simulink model "TimxAllConfigurations"  (R2018b)
settings: Solver=FixedStepDiscrete  StartTime=0.0  StopTime=10.0  RelTol=1e-3
libraries: TIMERS_Lib x7, STM32_Config_Lib x1
settings Model: Creator=fenard1  LastModifiedBy=fenard1
settings OptimizationCC: DefaultParameterBehavior=Inlined  DefaultUnderspecifiedDataType=single  EnhancedBackFolding=on  PassReuseOutputArgsAs=Individual arguments  OptimizeBlockOrder=speed  DifferentSizesBufferReuse=on  OptimizationCustomize=off
settings DebuggingCC: ParameterTunabilityLossMsg=error  UniqueDataStoreMsg=error  StrictBusMsg=ErrorOnBusTreatedAsVector  SFUndirectedBroadcastEventsDiag=error
settings HardwareCC: ProdBitPerPointer=32  ProdBitPerSizeT=32  ProdBitPerPtrDiffT=32  ProdLargestAtomicInteger=Integer  ProdWordSize=32  ProdHWDeviceType=STM32CortexM
settings SFSimCC: CompileTimeRecursionLimit=0  EnableRuntimeRecursion=off  MATLABDynamicMemAlloc=off
settings RTWCC: SystemTargetFile=stm32.tlc  TemplateMakefile=stm32.tmf  Description=stm32 (Embedded Target)  GenerateReport=on  IncludeHyperlinkInReport=on
settings CodeAppCC: ForceParamTrailComments=on  IgnoreCustomStorageClasses=off  OperatorAnnotations=on  SimulinkDataObjDesc=on  SFDataObjDesc=on  CustomSymbolStrType=$N$R$M  SimulinkBlockComments=off
settings STFCustomTargetCC: TargetLangStandard=C99 (ISO)  MultiwordLength=256  ParMdlRefBuildCompliant=on  IncludeMdlTerminateFcn=off  CombineOutputUpdateFcns=on  ERTCustomFileBanners=on  SupportComplex=off  SupportContinuousTime=off  SupportNonInlinedSFcns=off  RemoveResetFunc=on  ParenthesesLevel=Maximum  CastingMode=Standards  MATLABClassNameForMDSCustomization=Simulink.SoftwareTarget.ERTCustomization  SystemTargetFile=stm32.tlc
settings ERTTargetCC: TargetLangStandard=C99 (ISO)  CompOptLevelCompliant=off  ConcurrentExecutionCompliant=off  IncludeMdlTerminateFcn=off  SupportComplex=off  ParenthesesLevel=Maximum  CastingMode=Standards  ModelStepFunctionPrototypeControlCompliant=off  CPPClassGenCompliant=off  UseToolchainInfoCompliant=off  ExtModeStaticAllocSize=256  ExtModeMexArgs=0,1,115200,10  InlinedParameterPlacement=NonHierarchical  ERTSrcFileBannerTemplate=sourceFileTemplate.cgt  ERTHdrFileBannerTemplate=sourceFileTemplate.cgt  ERTDataSrcFileTemplate=sourceFileTemplate.cgt  ERTDataHdrFileTemplate=sourceFileTemplate.cgt  ERTCustomFileTemplate=customRoutineProcess.tlc  EnableSignedLeftShifts=off  EnableSignedRightShifts=off

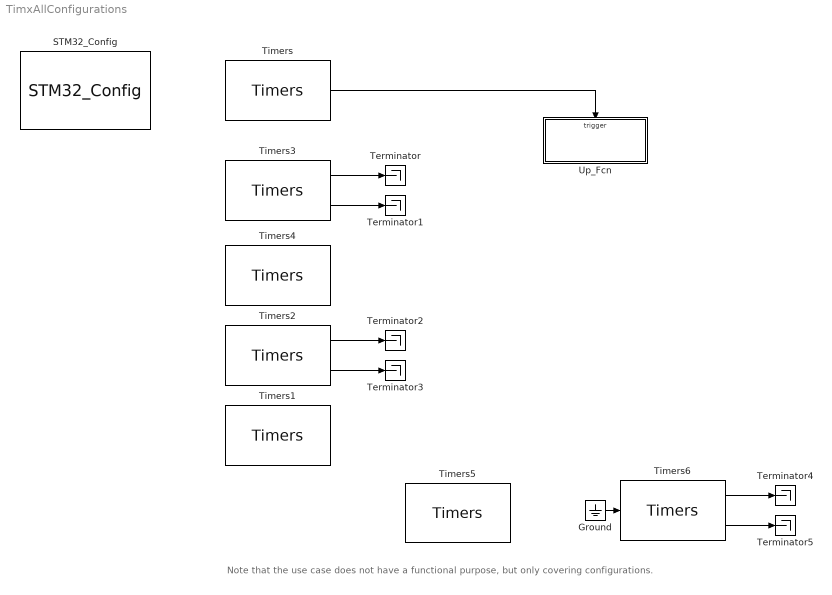
== system TimxAllConfigurations ==
  note: Note that the use case does not have a functional purpose, but only covering configurations.
  Ground : Ground
  STM32_Config : STM32_Config_Lib/STM32_Config  Priority=0  Project_Path=.\  Config_File=TimxAllConfigurations.ioc  MCU_Name=STM32F429ZITx
      settings: SourceProductName=Target Support Package - STM32 Adapter
  Terminator{,1..5} (6 alike) : Terminator
  Timers : TIMERS_Lib/Timers  currentTIM=TIM1  TIM_Name=TIM1  sysUsingTimer=on  TIM_APBClock=180000000  TIM_Set_Clk=off  TIM_Prescaler=2  TIM_Clock=60000000.00  Variable_frequency=off  TIM_Set_OutFreq=off  TIM_ARR=1  Output_frequency=60000000.00  Repetition_counter=0  TIM_Mode=Up  TIM_DMA=none  TIM_IRQ=on  TIM_IRQ_ONLY=off  TIM_UP=on  TIM_TRG=off  TIM_COM=off  TIM_BRK=off  NbTIM=7  CH1_enable=off  CH1N_enable=off  CH1_type=Input_Capture  CH1_DMA=off  CH1_int=off  CH1_edge=Rising  CH1_div=1  CH1_variable_duty=off  CH1_set_pulse=off  CH1_output_duty=0.00  CH1_pulse=0  CH2_enable=on  CH2N_enable=off  CH2_type=Output_Comp  CH2_DMA=off  CH2_int=off  CH2_edge=Rising  CH2_div=1  CH2_variable_duty=off  CH2_set_pulse=off  CH2_output_duty=0.00  CH2_pulse=0  CH3_enable=on  CH3N_enable=on  CH3_type=Output_Comp  CH3_DMA=off  CH3_int=off  CH3_edge=Rising  CH3_div=1  CH3_variable_duty=off  CH3_set_pulse=off  CH3_output_duty=0.00  CH3_pulse=0  CH4_enable=off  CH4N_enable=off  CH4_type=Input_Capture  CH4_DMA=off  CH4_int=off  CH4_edge=Rising  CH4_div=1  CH4_variable_duty=off  CH4_set_pulse=off  CH4_output_duty=0.00  CH4_pulse=0
      settings: SourceProductName=Target Support Package - STM32 Adapter
  Timers1 : TIMERS_Lib/Timers  currentTIM=TIM5  TIM_Name=TIM5  sysUsingTimer=on  TIM_APBClock=90000000  TIM_Set_Clk=off  TIM_Prescaler=0  TIM_Clock=90000000.00  Variable_frequency=off  TIM_Set_OutFreq=off  TIM_ARR=1  Output_frequency=90000000.00  Repetition_counter=0  TIM_Mode=Up  TIM_DMA=none  TIM_IRQ=off  TIM_IRQ_ONLY=on  TIM_UP=off  TIM_TRG=off  TIM_COM=off  TIM_BRK=off  NbTIM=7  CH1_enable=off  CH1N_enable=off  CH1_type=Input_Capture  CH1_DMA=off  CH1_int=off  CH1_edge=Rising  CH1_div=1  CH1_variable_duty=off  CH1_set_pulse=off  CH1_output_duty=0.00  CH1_pulse=0  CH2_enable=on  CH2N_enable=off  CH2_type=Input_Capture  CH2_DMA=off  CH2_int=off  CH2_edge=Rising  CH2_div=1  CH2_variable_duty=off  CH2_set_pulse=off  CH2_output_duty=0.00  CH2_pulse=0  CH3_enable=on  CH3N_enable=off  CH3_type=Output_Comp  CH3_DMA=off  CH3_int=off  CH3_edge=Rising  CH3_div=1  CH3_variable_duty=off  CH3_set_pulse=off  CH3_output_duty=0.00  CH3_pulse=0  CH4_enable=on  CH4N_enable=off  CH4_type=Output_Forced  CH4_DMA=off  CH4_int=off  CH4_edge=Rising  CH4_div=1  CH4_variable_duty=off  CH4_set_pulse=off  CH4_output_duty=0.00  CH4_pulse=0
      settings: SourceProductName=Target Support Package - STM32 Adapter
  Timers2 : TIMERS_Lib/Timers  currentTIM=TIM4  TIM_Name=TIM4  sysUsingTimer=on  TIM_APBClock=90000000  TIM_Set_Clk=off  TIM_Prescaler=0  TIM_Clock=90000000.00  Variable_frequency=off  TIM_Set_OutFreq=off  TIM_ARR=1  Output_frequency=90000000.00  Repetition_counter=0  TIM_Mode=Up  TIM_DMA=none  TIM_IRQ=off  TIM_IRQ_ONLY=off  TIM_UP=off  TIM_TRG=off  TIM_COM=off  TIM_BRK=off  NbTIM=7  CH1_enable=on  CH1N_enable=off  CH1_type=Input_Capture  CH1_DMA=off  CH1_int=off  CH1_edge=Rising  CH1_div=1  CH1_variable_duty=off  CH1_set_pulse=off  CH1_output_duty=0.00  CH1_pulse=0  CH2_enable=on  CH2N_enable=off  CH2_type=Output_Comp  CH2_DMA=off  CH2_int=off  CH2_edge=Rising  CH2_div=1  CH2_variable_duty=off  CH2_set_pulse=off  CH2_output_duty=0.00  CH2_pulse=0  CH3_enable=on  CH3N_enable=off  CH3_type=Output_PWM  CH3_DMA=off  CH3_int=off  CH3_edge=Rising  CH3_div=1  CH3_variable_duty=off  CH3_set_pulse=off  CH3_output_duty=0.00  CH3_pulse=0  CH4_enable=on  CH4N_enable=off  CH4_type=Output_Forced  CH4_DMA=off  CH4_int=off  CH4_edge=Rising  CH4_div=1  CH4_variable_duty=off  CH4_set_pulse=off  CH4_output_duty=0.00  CH4_pulse=0
      settings: SourceProductName=Target Support Package - STM32 Adapter
  Timers3 : TIMERS_Lib/Timers  currentTIM=TIM2  TIM_Name=TIM2  sysUsingTimer=on  TIM_APBClock=90000000  TIM_Set_Clk=off  TIM_Prescaler=0  TIM_Clock=90000000.00  Variable_frequency=off  TIM_Set_OutFreq=off  TIM_ARR=1  Output_frequency=90000000.00  Repetition_counter=0  TIM_Mode=Down  TIM_DMA=none  TIM_IRQ=off  TIM_IRQ_ONLY=off  TIM_UP=off  TIM_TRG=off  TIM_COM=off  TIM_BRK=off  NbTIM=7  CH1_enable=on  CH1N_enable=off  CH1_type=Input_Capture  CH1_DMA=off  CH1_int=off  CH1_edge=Rising  CH1_div=1  CH1_variable_duty=off  CH1_set_pulse=off  CH1_output_duty=0.00  CH1_pulse=0  CH2_enable=off  CH2N_enable=off  CH2_type=Output_PWM  CH2_DMA=off  CH2_int=off  CH2_edge=Rising  CH2_div=1  CH2_variable_duty=off  CH2_set_pulse=off  CH2_output_duty=0.00  CH2_pulse=0  CH3_enable=off  CH3N_enable=off  CH3_type=Output_Forced  CH3_DMA=off  CH3_int=off  CH3_edge=Rising  CH3_div=1  CH3_variable_duty=off  CH3_set_pulse=off  CH3_output_duty=0.00  CH3_pulse=0  CH4_enable=off  CH4N_enable=off  CH4_type=Unknown  CH4_DMA=off  CH4_int=off  CH4_edge=Rising  CH4_div=1  CH4_variable_duty=off  CH4_set_pulse=off  CH4_output_duty=0.00  CH4_pulse=0
      settings: SourceProductName=Target Support Package - STM32 Adapter
  Timers4 : TIMERS_Lib/Timers  currentTIM=TIM3  TIM_Name=TIM3  sysUsingTimer=on  TIM_APBClock=90000000  TIM_Set_Clk=off  TIM_Prescaler=0  TIM_Clock=90000000.00  Variable_frequency=off  TIM_Set_OutFreq=off  TIM_ARR=1  Output_frequency=90000000.00  Repetition_counter=0  TIM_Mode=Center_Aligned_1  TIM_DMA=none  TIM_IRQ=off  TIM_IRQ_ONLY=off  TIM_UP=off  TIM_TRG=off  TIM_COM=off  TIM_BRK=off  NbTIM=7  CH1_enable=off  CH1N_enable=off  CH1_type=Output_Forced  CH1_DMA=off  CH1_int=off  CH1_edge=Rising  CH1_div=1  CH1_variable_duty=off  CH1_set_pulse=off  CH1_output_duty=0.00  CH1_pulse=0  CH2_enable=on  CH2N_enable=off  CH2_type=Output_PWM  CH2_DMA=off  CH2_int=off  CH2_edge=Rising  CH2_div=1  CH2_variable_duty=off  CH2_set_pulse=off  CH2_output_duty=0.00  CH2_pulse=0  CH3_enable=on  CH3N_enable=off  CH3_type=Output_Forced  CH3_DMA=off  CH3_int=off  CH3_edge=Rising  CH3_div=1  CH3_variable_duty=off  CH3_set_pulse=off  CH3_output_duty=0.00  CH3_pulse=0  CH4_enable=off  CH4N_enable=off  CH4_type=Output_PWM  CH4_DMA=off  CH4_int=off  CH4_edge=Rising  CH4_div=1  CH4_variable_duty=off  CH4_set_pulse=off  CH4_output_duty=0.00  CH4_pulse=0
      settings: SourceProductName=Target Support Package - STM32 Adapter
  Timers5 : TIMERS_Lib/Timers  currentTIM=TIM7  TIM_Name=TIM7  sysUsingTimer=on  TIM_APBClock=90000000  TIM_Set_Clk=off  TIM_Prescaler=0  TIM_Clock=90000000.00  Variable_frequency=off  TIM_Set_OutFreq=off  TIM_ARR=1  Output_frequency=90000000.00  Repetition_counter=0  TIM_Mode=Up  TIM_DMA=none  TIM_IRQ=off  TIM_IRQ_ONLY=on  TIM_UP=off  TIM_TRG=off  TIM_COM=off  TIM_BRK=off  NbTIM=7  CH1_enable=off  CH1N_enable=off  CH1_type=Unknown  CH1_DMA=off  CH1_int=off  CH1_edge=Rising  CH1_div=1  CH1_variable_duty=off  CH1_set_pulse=off  CH1_output_duty=0.00  CH1_pulse=0  CH2_enable=off  CH2N_enable=off  CH2_type=Unknown  CH2_DMA=off  CH2_int=off  CH2_edge=Rising  CH2_div=1  CH2_variable_duty=off  CH2_set_pulse=off  CH2_output_duty=0.00  CH2_pulse=0  CH3_enable=off  CH3N_enable=off  CH3_type=Unknown  CH3_DMA=off  CH3_int=off  CH3_edge=Rising  CH3_div=1  CH3_variable_duty=off  CH3_set_pulse=off  CH3_output_duty=0.00  CH3_pulse=0  CH4_enable=off  CH4N_enable=off  CH4_type=Unknown  CH4_DMA=off  CH4_int=off  CH4_edge=Rising  CH4_div=1  CH4_variable_duty=off  CH4_set_pulse=off  CH4_output_duty=0.00  CH4_pulse=0
      settings: SourceProductName=Target Support Package - STM32 Adapter
  Timers6 : TIMERS_Lib/Timers  currentTIM=TIM8  TIM_Name=TIM8  sysUsingTimer=on  TIM_APBClock=180000000  TIM_Set_Clk=off  TIM_Prescaler=0  TIM_Clock=180000000.00  Variable_frequency=off  TIM_Set_OutFreq=off  TIM_ARR=1399  Output_frequency=128663.33  Repetition_counter=0  TIM_Mode=Up  TIM_DMA=none  TIM_IRQ=off  TIM_IRQ_ONLY=off  TIM_UP=off  TIM_TRG=off  TIM_COM=off  TIM_BRK=off  NbTIM=7  CH1_enable=on  CH1N_enable=off  CH1_type=Input_Encoder  CH1_DMA=off  CH1_int=off  CH1_edge=Rising  CH1_div=1  CH1_variable_duty=off  CH1_set_pulse=off  CH1_output_duty=0.00  CH1_pulse=0  CH2_enable=on  CH2N_enable=off  CH2_type=Input_Encoder  CH2_DMA=off  CH2_int=off  CH2_edge=Rising  CH2_div=1  CH2_variable_duty=off  CH2_set_pulse=off  CH2_output_duty=0.00  CH2_pulse=0  CH3_enable=off  CH3N_enable=off  CH3_type=Unknown  CH3_DMA=off  CH3_int=off  CH3_edge=Rising  CH3_div=1  CH3_variable_duty=off  CH3_set_pulse=off  CH3_output_duty=0.00  CH3_pulse=0  CH4_enable=off  CH4N_enable=off  CH4_type=Unknown  CH4_DMA=off  CH4_int=off  CH4_edge=Rising  CH4_div=1  CH4_variable_duty=off  CH4_set_pulse=off  CH4_output_duty=0.00  CH4_pulse=0
      settings: SourceProductName=Target Support Package - STM32 Adapter
  "Up_Fcn " : Subsystem  TreatAsAtomicUnit=on
  wires:
  Timers/1 -> "Up_Fcn "/Trigger
  Timers3/1 -> Terminator/1
  Timers3/2 -> Terminator1/1
  Timers2/1 -> Terminator2/1
  Timers2/2 -> Terminator3/1
  Timers6/1 -> Terminator4/1
  Timers6/2 -> Terminator5/1
  Ground/1 -> Timers6/1

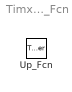
== system TimxAllConfigurations/Up_Fcn  ==
  Up_Fcn : TriggerPort  TriggerType=function-call  VariantControl=Variant
